simulink model "PD_controller_by_Blocks"  (R2022b)
settings: Solver=VariableStepAuto  StartTime=0.0  StopTime=20  RelTol=1e-3
values from neighbouring files (symbols this model uses):
  J_L = 1    [Parameters.m]
  K_b = 0.05    [Parameters.m]
  K_t = 0.05    [Parameters.m]
  L_a = 500*10^-6    (= 0.0005)    [Parameters.m]
  N1 = 1    [Parameters.m]
  N2 = 50    [Parameters.m]
  R_a = 5    [Parameters.m]
settings Model: Creator=عالم الكمبيوتر  LastModifiedBy=عالم الكمبيوتر

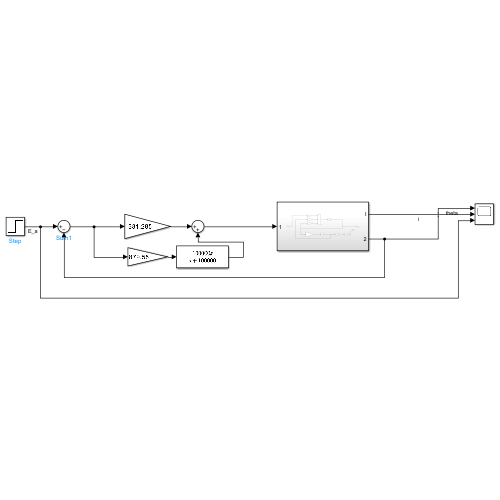
[thumbnail: Simulink's stored preview of the top-level diagram]
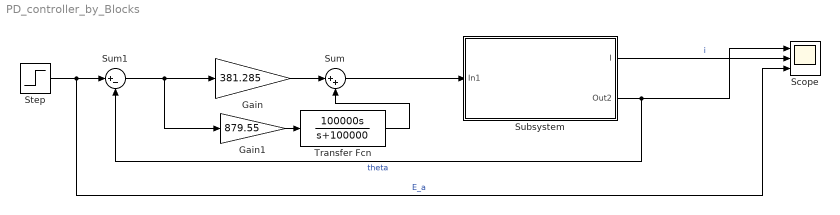
== system PD_controller_by_Blocks ==
  Gain : Gain  Gain=381.285
  Gain1 : Gain  Gain=879.55
  Scope : Scope  NumInputPorts=3
  Step : Step  SampleTime=0
  Subsystem : Subsystem
  Sum : Sum  Inputs=|++
  Sum1 : Sum  Inputs=|+-
  Transfer Fcn : TransferFcn  Numerator=[100000 0]  Denominator=[1 100000]
  wires:
  Step/1 -> Scope/3, Sum1/1  "E_a"
  Subsystem/2(Out2) -> Scope/1, Sum1/2  "theta"
  Sum/1 -> Subsystem/1(In1)
  Subsystem/1(I) -> Scope/2  "i"
  Gain/1 -> Sum/1
  Sum1/1 -> Gain1/1, Gain/1
  Gain1/1 -> Transfer Fcn/1
  Transfer Fcn/1 -> Sum/2

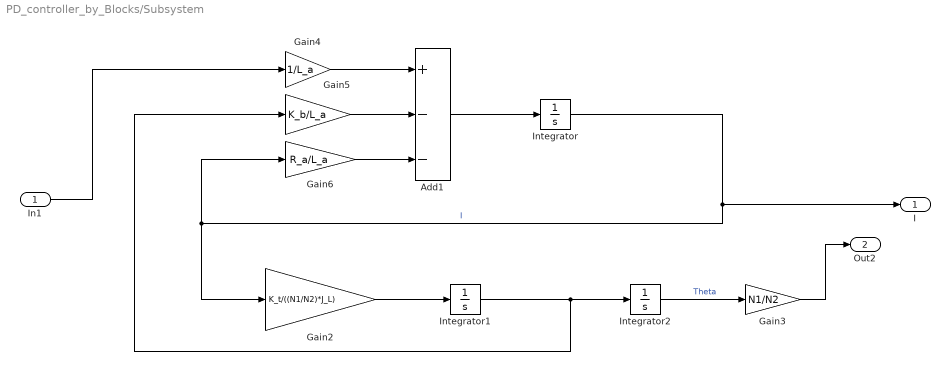
== system PD_controller_by_Blocks/Subsystem ==
  In1 : Inport
  Add1 : Sum  Inputs=+--
  Gain2 : Gain  Gain=K_t/((N1/N2)*J_L)
  Gain3 : Gain  Gain=N1/N2
  Gain4 : Gain  Gain=1/L_a
  Gain5 : Gain  Gain=K_b/L_a
  Gain6 : Gain  Gain=R_a/L_a
  Integrator : Integrator
  Integrator1 : Integrator
  Integrator2 : Integrator
  I : Outport
  Out2 : Outport  Port=2
  wires:
  Gain4/1 -> Add1/1
  Integrator/1 -> I/1, Gain6/1, Gain2/1  "I"
  Integrator2/1 -> Gain3/1  "Theta"
  Gain6/1 -> Add1/3
  Add1/1 -> Integrator/1
  Integrator1/1 -> Gain5/1, Integrator2/1
  Gain2/1 -> Integrator1/1
  Gain5/1 -> Add1/2
  In1/1 -> Gain4/1
  Gain3/1 -> Out2/1
